simulink model "rhszero_2dof"  (R2014b)
settings: Solver=ode45  StartTime=0.0  StopTime=10.0  RelTol=1e-3
values from neighbouring files (symbols this model uses):
  a = -1    [abs_spring18.m]    (also in hw_tank_simulink_pid_tuning.m = 2.085; pmsm_fall19.m = 0.427011494253; rhszero_variables.m = 4; tanker_yaw_lead_zero.m)
settings Model: Creator=kjartan  LastModifiedBy=kjartan

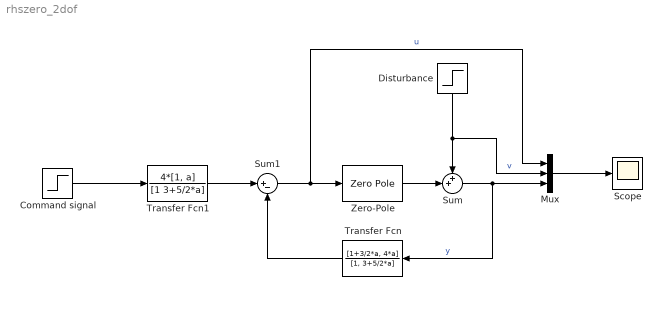
== system rhszero_2dof ==
  Command signal : Step  Time=0  SampleTime=0
  Disturbance : Step  Time=5  SampleTime=0
  Mux : Mux  Inputs=3
  Scope : Scope
      settings: ShowLegends=on
  Sum : Sum  Inputs=++|
  Sum1 : Sum  Inputs=|+-
  Transfer Fcn : TransferFcn  Numerator=[1+3/2*a, 4*a]  Denominator=[1, 3+5/2*a]
  Transfer Fcn1 : TransferFcn  Numerator=4*[1, a]  Denominator=[1 3+5/2*a]
  Zero-Pole : ZeroPole  Zeros=[2]  Poles=[0, -2]  Gain=[-1]
  wires:
  Sum/1 -> Transfer Fcn/1, Mux/3  "y"
  Zero-Pole/1 -> Sum/2
  Mux/1 -> Scope/1
  Command signal/1 -> Transfer Fcn1/1
  Disturbance/1 -> Mux/2, Sum/1  "v"
  Sum1/1 -> Mux/1, Zero-Pole/1  "u"
  Transfer Fcn/1 -> Sum1/2
  Transfer Fcn1/1 -> Sum1/1
